simulink model "Requirement_table_and_model"  (R2022b)
settings: Solver=FixedStepAuto  StartTime=0.0  StopTime=10.0  FixedStep=1e-3  RelTol=1e-3  EnableMultiTasking=on
model workspace (MAT data in the model file):
  ATR_CMP_DETECT = canlib.Parameter
  ATR_CMP_DETECT.DataType = 'boolean'
  ATR_CMP_DETECT.Complexity = 'real'
  ATR_CMP_DETECT.Dimensions = [0 0]
  ATR_GND_CTRL = canlib.Parameter
  ATR_GND_CTRL.DataType = 'auto'
  ATR_GND_CTRL.Complexity = 'real'
  ATR_GND_CTRL.Dimensions = [0 0]
  ATR_PACE_CTRL = SimulinkDemos.Signal
  ATR_PACE_CTRL.DataType = 'auto'
  ATR_PACE_CTRL.Dimensions = -1
  ATR_PACE_CTRL.DimensionsMode = 'auto'
  ATR_PACE_CTRL.Complexity = 'auto'
  ATR_PACE_CTRL.SampleTime = -1
  ATR_PACE_CTRL.SamplingMode = 'auto'
  ATR_PULSE_WIDTH = SimulinkDemos.Signal
  ATR_PULSE_WIDTH.DataType = 'auto'
  ATR_PULSE_WIDTH.Dimensions = -1
  ATR_PULSE_WIDTH.DimensionsMode = 'auto'
  ATR_PULSE_WIDTH.Complexity = 'auto'
  ATR_PULSE_WIDTH.SampleTime = -1
  ATR_PULSE_WIDTH.SamplingMode = 'auto'
  ATR_REF = SimulinkDemos.Signal
  ATR_REF.DataType = 'auto'
  ATR_REF.Dimensions = -1
  ATR_REF.DimensionsMode = 'auto'
  ATR_REF.Complexity = 'auto'
  ATR_REF.SampleTime = -1
  ATR_REF.SamplingMode = 'auto'
  FRONTEND_CTRL = SimulinkDemos.Signal
  FRONTEND_CTRL.DataType = 'auto'
  FRONTEND_CTRL.Dimensions = -1
  FRONTEND_CTRL.DimensionsMode = 'auto'
  FRONTEND_CTRL.Complexity = 'auto'
  FRONTEND_CTRL.SampleTime = -1
  FRONTEND_CTRL.SamplingMode = 'auto'
  LRL = SimulinkDemos.Signal
  LRL.DataType = 'auto'
  LRL.Dimensions = -1
  LRL.DimensionsMode = 'auto'
  LRL.Complexity = 'auto'
  LRL.SampleTime = -1
  LRL.SamplingMode = 'auto'
  PACE_CHARGE_CTRL = SimulinkDemos.Signal
  PACE_CHARGE_CTRL.DataType = 'auto'
  PACE_CHARGE_CTRL.Dimensions = -1
  PACE_CHARGE_CTRL.DimensionsMode = 'auto'
  PACE_CHARGE_CTRL.Complexity = 'auto'
  PACE_CHARGE_CTRL.SampleTime = -1
  PACE_CHARGE_CTRL.SamplingMode = 'auto'
  PACE_GND_CTRL = SimulinkDemos.Signal
  PACE_GND_CTRL.DataType = 'auto'
  PACE_GND_CTRL.Dimensions = -1
  PACE_GND_CTRL.DimensionsMode = 'auto'
  PACE_GND_CTRL.Complexity = 'auto'
  PACE_GND_CTRL.SampleTime = -1
  PACE_GND_CTRL.SamplingMode = 'auto'
  VENT_CMP_DETECT = SimulinkDemos.Signal
  VENT_CMP_DETECT.DataType = 'auto'
  VENT_CMP_DETECT.Dimensions = -1
  VENT_CMP_DETECT.DimensionsMode = 'auto'
  VENT_CMP_DETECT.Complexity = 'auto'
  VENT_CMP_DETECT.SampleTime = -1
  VENT_CMP_DETECT.SamplingMode = 'auto'
  VENT_GND_CTRL = SimulinkDemos.Signal
  VENT_GND_CTRL.DataType = 'auto'
  VENT_GND_CTRL.Dimensions = -1
  VENT_GND_CTRL.DimensionsMode = 'auto'
  VENT_GND_CTRL.Complexity = 'auto'
  VENT_GND_CTRL.SampleTime = -1
  VENT_GND_CTRL.SamplingMode = 'auto'
  VENT_PACE_CTRL = SimulinkDemos.Signal
  VENT_PACE_CTRL.DataType = 'auto'
  VENT_PACE_CTRL.Dimensions = -1
  VENT_PACE_CTRL.DimensionsMode = 'auto'
  VENT_PACE_CTRL.Complexity = 'auto'
  VENT_PACE_CTRL.SampleTime = -1
  VENT_PACE_CTRL.SamplingMode = 'auto'
  VENT_PULSE_WIDTH = SimulinkDemos.Signal
  VENT_PULSE_WIDTH.DataType = 'auto'
  VENT_PULSE_WIDTH.Dimensions = -1
  VENT_PULSE_WIDTH.DimensionsMode = 'auto'
  VENT_PULSE_WIDTH.Complexity = 'auto'
  VENT_PULSE_WIDTH.SampleTime = -1
  VENT_PULSE_WIDTH.SamplingMode = 'auto'
  VENT_REF = SimulinkDemos.Signal
  VENT_REF.DataType = 'auto'
  VENT_REF.Dimensions = -1
  VENT_REF.DimensionsMode = 'auto'
  VENT_REF.Complexity = 'auto'
  VENT_REF.SampleTime = -1
  VENT_REF.SamplingMode = 'auto'
  Z_ATR_CTRL = SimulinkDemos.Signal
  Z_ATR_CTRL.DataType = 'auto'
  Z_ATR_CTRL.Dimensions = -1
  Z_ATR_CTRL.DimensionsMode = 'auto'
  Z_ATR_CTRL.Complexity = 'auto'
  Z_ATR_CTRL.SampleTime = -1
  Z_ATR_CTRL.SamplingMode = 'auto'
  Z_VENT_CTRL = SimulinkDemos.Signal
  Z_VENT_CTRL.DataType = 'auto'
  Z_VENT_CTRL.Dimensions = -1
  Z_VENT_CTRL.DimensionsMode = 'auto'
  Z_VENT_CTRL.Complexity = 'auto'
  Z_VENT_CTRL.SampleTime = -1
  Z_VENT_CTRL.SamplingMode = 'auto'
undefined symbols (not defined in the file): D0, D1, D10, D11, D12, D13, D2, D3, D4, D5, D6, D7, D8, D9, PTA0, PTA1, PTA2, PTB23, PTB9, PTC16, PTC17, PTC2, PTC3, PTC4, PTD0, PTD1, PTD2, PTD3
libraries: frdmk64flib x14
settings Model: ExtModeTrigDuration=5  Creator=clara  LastModifiedBy=dinghao
settings OptimizationCC: EnhancedBackFolding=on  PassReuseOutputArgsAs=Individual arguments  ZeroExternalMemoryAtStartup=off  ZeroInternalMemoryAtStartup=off  MaxStackSize=64  OptimizeBlockOrder=speed  DifferentSizesBufferReuse=on  OptimizationCustomize=off  EfficientTunableParamExpr=on
settings DebuggingCC: ParameterTunabilityLossMsg=error  SFUnusedDataAndEventsDiag=none
settings HardwareCC: ProdBitPerPointer=32  ProdBitPerSizeT=32  ProdBitPerPtrDiffT=32  ProdLargestAtomicInteger=Long  ProdLargestAtomicFloat=Double  ProdWordSize=32  ProdHWDeviceType=ARM Compatible->ARM Cortex
settings ModelReferenceCC: EnableRefExpFcnMdlSchedulingChecks=on
settings SFSimCC: MATLABDynamicMemAlloc=off
settings RTWCC: Description=Embedded Coder  SystemTargetFile=ert.tlc  HardwareBoard=NXP FRDM-K64F  TLCOptions="-aInlineSetEventsForThisBaseRateFcn=TLC_FALSE -aSuppressMultiTaskScheduler=TLC_FALSE  -aRateBasedStepFcn=0"  TemplateMakefile=ert_default_tmf  Toolchain=GNU Tools for ARM Embedded Processors
settings CodeAppCC: ForceParamTrailComments=on  IgnoreCustomStorageClasses=off  OperatorAnnotations=on  SimulinkDataObjDesc=on  SFDataObjDesc=on  InsertBlockDesc=on
settings ERTTargetCC: ExtModeTransport=4  ExtModeMexFile=sendToCommService

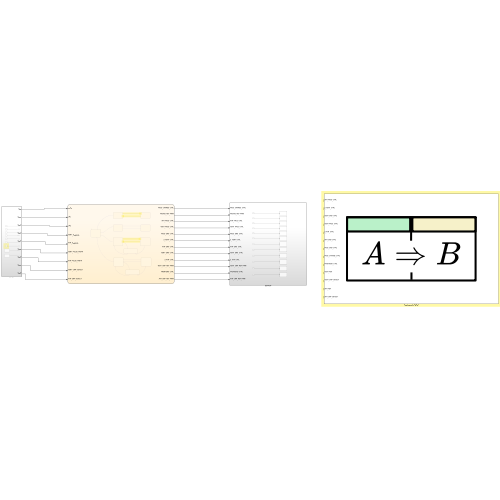
[thumbnail: Simulink's stored preview of the top-level diagram]
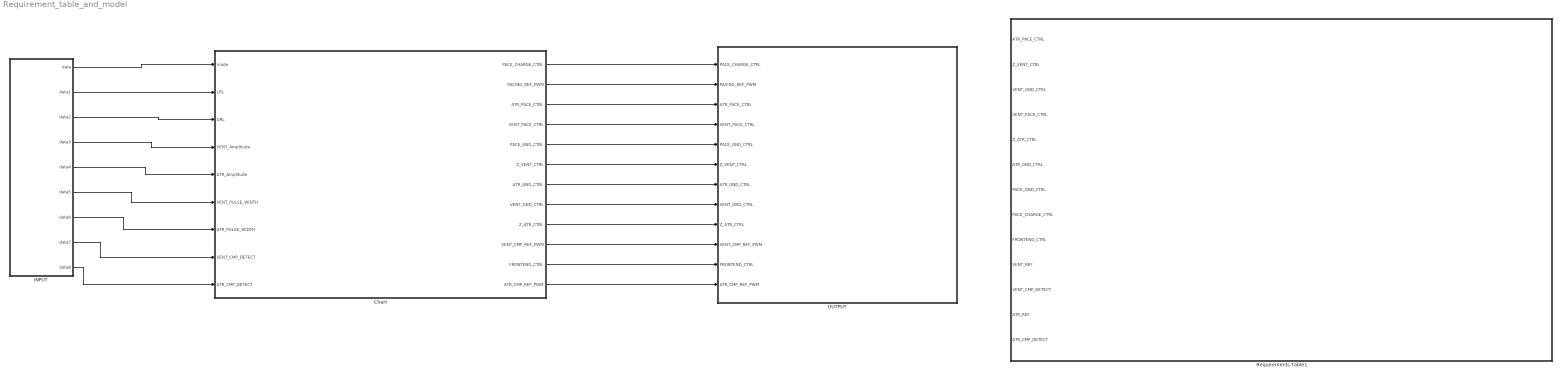
== system Requirement_table_and_model ==
  Chart : Stateflow chart  TreatAsAtomicUnit=on
      settings: PortSchema="{\"entries\":[{\"content\":{\"sides\":[{\"content\":{\"connectorIds\":[\"In9\",\"In1\",\"In6\",\"In2\",\"In3\",\"In4\",\"In5\",\"In7\",\"In8\"]},\"type\":\"ConnectorPlacement.EquallySpacedRectSide\",\"uuid\":\"411cfc43-89c3-4653-9fab-0da98be593d3\"},{\"content\":{\"connectorIds\":[\"Out1\",\"Out2\",\"Out3\",\"Out4\",\"Out5\",\"Out6\",\"Out7\",\"Out8\",\"Out9\",\"Out10\",\"Out11\",\"Out12\"],\"side\":\"RIGHT\"},\"type\":\"ConnectorPlacement.EquallySpacedRectSide\",\"uuid\":\"ad1683f7-26aa-4767-b656-f3b731cb8235\"},{\"content\":{\"connectorIds\":[],\"side\":\"TOP\"},\"type\":\"ConnectorPlacement.EquallySpacedRectSide\",\"uuid\":\"fbccba07-c1cc-4c9f-8e56-0bdfb6912bb8\"},{\"content\":{\"connectorIds\":[],\"side\":\"BOTTOM\"},\"type\":\"ConnectorPlacement.EquallySpacedRectSide\",\"uuid\":\"36d5a70a-9c4d-4c73-b058-58220445b1e8\"}]},\"type\":\"ConnectorPlacement.EquallySpacedConnector\",\"uuid\":\"0c618a7f-9484-4de3-a6ac-3c8308721375\"}],\"packageUris\":[\"http://schema.mathworks.com/mf0/Connector/R2020b\"],\"version\":\"1.0\"}"
  "INPUT " : Subsystem
  OUTPUT : Subsystem
  Requirements Table1 : Requirements Table  TreatAsAtomicUnit=on
  wires:
  Chart/7(ATR_GND_CTRL) -> OUTPUT/7(ATR_GND_CTRL)
  Chart/3(ATR_PACE_CTRL) -> OUTPUT/3(ATR_PACE_CTRL)
  Chart/6(Z_VENT_CTRL) -> OUTPUT/6(Z_VENT_CTRL)
  Chart/8(VENT_GND_CTRL) -> OUTPUT/8(VENT_GND_CTRL)
  Chart/5(PACE_GND_CTRL) -> OUTPUT/5(PACE_GND_CTRL)
  Chart/9(Z_ATR_CTRL) -> OUTPUT/9(Z_ATR_CTRL)
  Chart/2(PACING_REF_PWM) -> OUTPUT/2(PACING_REF_PWM)
  Chart/1(PACE_CHARGE_CTRL) -> OUTPUT/1(PACE_CHARGE_CTRL)
  Chart/4(VENT_PACE_CTRL) -> OUTPUT/4(VENT_PACE_CTRL)
  Chart/11(FRONTEND_CTRL) -> OUTPUT/11(FRONTEND_CTRL)
  Chart/10(VENT_CMP_REF_PWM) -> OUTPUT/10(VENT_CMP_REF_PWM)
  "INPUT "/1(data) -> Chart/9(mode)
  "INPUT "/3(data2) -> Chart/6(URL)
  "INPUT "/4(data3) -> Chart/2(VENT_Amplitude)
  "INPUT "/5(data4) -> Chart/3(ATR_Amplitude)
  "INPUT "/6(data5) -> Chart/4(VENT_PULSE_WIDTH)
  "INPUT "/8(data7) -> Chart/7(VENT_CMP_DETECT)
  Chart/12(ATR_CMP_REF_PWM) -> OUTPUT/12(ATR_CMP_REF_PWM)
  "INPUT "/7(data6) -> Chart/5(ATR_PULSE_WIDTH)
  "INPUT "/2(data1) -> Chart/1(LRL)
  "INPUT "/9(data8) -> Chart/8(ATR_CMP_DETECT)

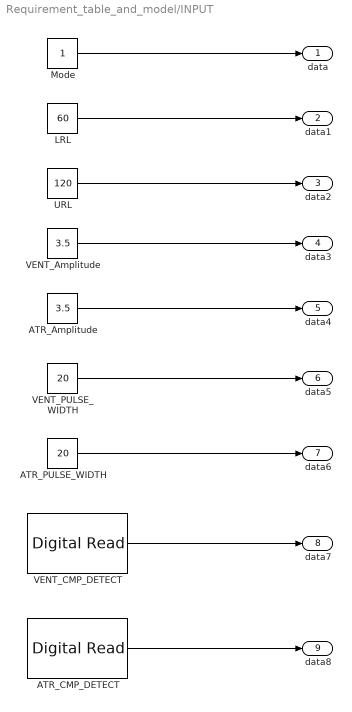
== system Requirement_table_and_model/INPUT  ==
  ATR_Amplitude : Constant  Value=3.5
  ATR_CMP_DETECT : frdmk64flib/Digital Read  Whichpin=PTC16 (D0)  SampleTime=-1
  ATR_PULSE_WIDTH : Constant  Value=20
  LRL : Constant  Value=60
  Mode : Constant
  URL : Constant  Value=120
  VENT_Amplitude : Constant  Value=3.5
  VENT_CMP_DETECT : frdmk64flib/Digital Read  Whichpin=PTC17 (D1)  SampleTime=-1
  VENT_PULSE_WIDTH : Constant  Value=20
  data : Outport
  data1 : Outport  Port=2
  data2 : Outport  Port=3
  data3 : Outport  Port=4
  data4 : Outport  Port=5
  data5 : Outport  Port=6
  data6 : Outport  Port=7
  data7 : Outport  Port=8
  data8 : Outport  Port=9
  wires:
  LRL/1 -> data1/1
  VENT_PULSE_WIDTH/1 -> data5/1
  VENT_Amplitude/1 -> data3/1
  URL/1 -> data2/1
  Mode/1 -> data/1
  ATR_Amplitude/1 -> data4/1
  ATR_PULSE_WIDTH/1 -> data6/1
  VENT_CMP_DETECT/1 -> data7/1
  ATR_CMP_DETECT/1 -> data8/1

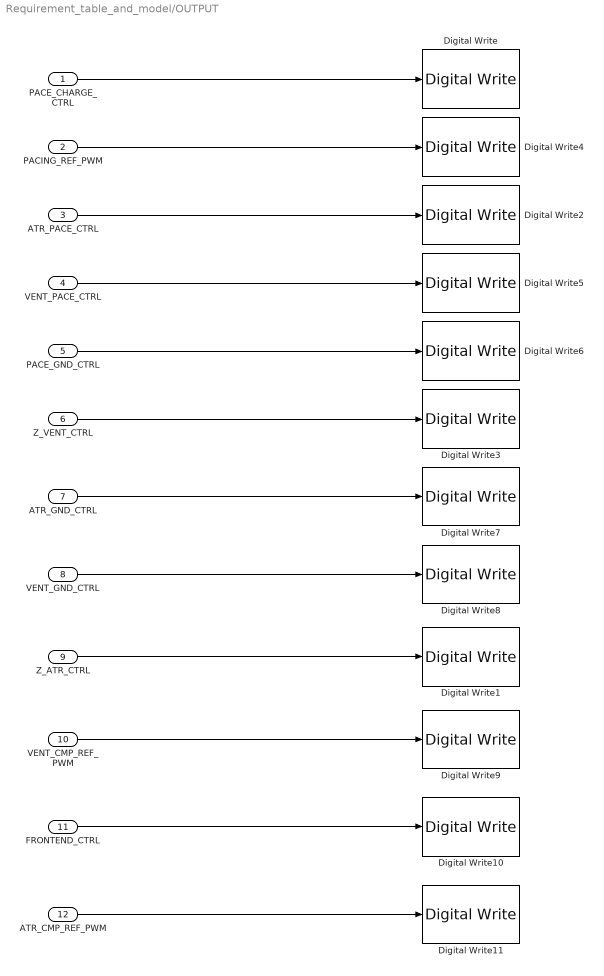
== system Requirement_table_and_model/OUTPUT ==
  PACE_CHARGE_CTRL : Inport
  PACING_REF_PWM : Inport  Port=2
  ATR_PACE_CTRL : Inport  Port=3
  VENT_PACE_CTRL : Inport  Port=4
  PACE_GND_CTRL : Inport  Port=5
  Z_VENT_CTRL : Inport  Port=6
  ATR_GND_CTRL : Inport  Port=7
  VENT_GND_CTRL : Inport  Port=8
  Z_ATR_CTRL : Inport  Port=9
  VENT_CMP_REF_PWM : Inport  Port=10
  FRONTEND_CTRL : Inport  Port=11
  ATR_CMP_REF_PWM : Inport  Port=12
  Digital Write : frdmk64flib/Digital Write  Whichpin=PTB9 (D2)
  Digital Write1 : frdmk64flib/Digital Write  Whichpin=PTB23 (D4)
  Digital Write10 : frdmk64flib/Digital Write  Whichpin=PTD1 (D13)
  Digital Write11 : frdmk64flib/Digital Write  Whichpin=PTC2 (D6)
  Digital Write2 : frdmk64flib/Digital Write  Whichpin=PTA0 (D8)
  Digital Write3 : frdmk64flib/Digital Write  Whichpin=PTC3 (D7)
  Digital Write4 : frdmk64flib/Digital Write  Whichpin=PTA2 (D5)
  Digital Write5 : frdmk64flib/Digital Write  Whichpin=PTC4 (D9)
  Digital Write6 : frdmk64flib/Digital Write  Whichpin=PTD0 (D10)
  Digital Write7 : frdmk64flib/Digital Write  Whichpin=PTD2 (D11)
  Digital Write8 : frdmk64flib/Digital Write  Whichpin=PTD3 (D12)
  Digital Write9 : frdmk64flib/Digital Write  Whichpin=PTA1 (D3)
  wires:
  PACE_CHARGE_CTRL/1 -> Digital Write/1
  PACING_REF_PWM/1 -> Digital Write4/1
  ATR_PACE_CTRL/1 -> Digital Write2/1
  VENT_PACE_CTRL/1 -> Digital Write5/1
  PACE_GND_CTRL/1 -> Digital Write6/1
  Z_VENT_CTRL/1 -> Digital Write3/1
  ATR_GND_CTRL/1 -> Digital Write7/1
  VENT_GND_CTRL/1 -> Digital Write8/1
  Z_ATR_CTRL/1 -> Digital Write1/1
  VENT_CMP_REF_PWM/1 -> Digital Write9/1
  FRONTEND_CTRL/1 -> Digital Write10/1
  ATR_CMP_REF_PWM/1 -> Digital Write11/1

== stateflow chart Requirement_table_and_model/Requirements Table1 ==
  (default) -> (junction 1073753366)
  (junction 1073753366) -> (junction 1073753367) : {
      | % SF_REQ_REV_07
      | }
  (junction 1073753367) -> (junction 1073753369) : {
      | % HEADER_ASSIGNMENTS
      |
      | }
  (junction 1073753369) -> (junction 1073753371) : {
      | % START_A_4
      | }
  (junction 1073753371) -> (junction 1073753373) : {
      | }
  (junction 1073753373) -> (junction 1073753375)
  (junction 1073753375) -> (junction 1073753377) : {
      | }
  (junction 1073753377) -> (junction 1073753379) : {
      | % END_A_4
      | }
  (junction 1073753379) -> (junction 1073753381) : {
      | % START_R_1
      | }
  (junction 1073753381) -> (junction 1073753383) : {
      | }
  (junction 1073753383) -> (junction 1073753385) : {
      |
      |
      |
      |
      |
      |
      |
      | }
  (junction 1073753385) -> (junction 1073753387) : {
      | }
  (junction 1073753387) -> (junction 1073753389) : {
      | % START_R_10
      | }
  (junction 1073753389) -> (junction 1073753391) : {
      | }
  (junction 1073753391) -> (junction 1073753393)
  (junction 1073753393) -> (junction 1073753395) [order 1] : [duration((prev(ATR_PACE_CTRL) == false) && (prev(PACE_CHARGE_CTRL) == true) && (prev(PACE_GND_CTRL) == true) && (prev(ATR_GND_CTRL) == true) && (prev(Z_ATR_CTRL) == false)) >= 60000/LRL-ATR_PULSE_WIDTH]
  (junction 1073753393) -> (junction 1073753401) [order 2]
  (junction 1073753395) -> (junction 1073753397) : {
      | ATR_PACE_CTRL == true
      | PACE_CHARGE_CTRL == false
      | PACE_GND_CTRL == true
      | ATR_GND_CTRL == false
      | Z_ATR_CTRL == false
      |
      |
      | }
  (junction 1073753397) -> (junction 1073753399) : {
      | }
  (junction 1073753399) -> (junction 1073753401)
  (junction 1073753401) -> (junction 1073753403)
  (junction 1073753403) -> (junction 1073753405) : {
      | % END_R_10
      | }
  (junction 1073753405) -> (junction 1073753407) : {
      | % START_R_13
      | }
  (junction 1073753407) -> (junction 1073753409) : {
      | }
  (junction 1073753409) -> (junction 1073753411)
  (junction 1073753411) -> (junction 1073753413) [order 1] : [duration((prev(ATR_PACE_CTRL) == true) && (prev(PACE_CHARGE_CTRL)== false) && (prev(PACE_GND_CTRL) == true) && (prev(ATR_GND_CTRL) == false) && (prev(Z_ATR_CTRL) == false)) >= ATR_PULSE_WIDTH]
  (junction 1073753411) -> (junction 1073753419) [order 2]
  (junction 1073753413) -> (junction 1073753415) : {
      | ATR_PACE_CTRL == false
      | PACE_CHARGE_CTRL == true
      | PACE_GND_CTRL == true
      | ATR_GND_CTRL == true
      | Z_ATR_CTRL == false
      |
      |
      | }
  (junction 1073753415) -> (junction 1073753417) : {
      | }
  (junction 1073753417) -> (junction 1073753419)
  (junction 1073753419) -> (junction 1073753421)
  (junction 1073753421) -> (junction 1073753423) : {
      | % END_R_13
      | }
  (junction 1073753423) -> (junction 1073753425) : {
      | % END_R_1
      | }
  (junction 1073753425) -> (junction 1073753427) : {
      | % START_R_16
      | }
  (junction 1073753427) -> (junction 1073753429) : {
      | }
  (junction 1073753429) -> (junction 1073753431) : {
      |
      |
      |
      |
      |
      |
      |
      | }
  (junction 1073753431) -> (junction 1073753433) : {
      | }
  (junction 1073753433) -> (junction 1073753435) : {
      | % START_R_19
      | }
  (junction 1073753435) -> (junction 1073753437) : {
      | }
  (junction 1073753437) -> (junction 1073753439)
  (junction 1073753439) -> (junction 1073753441) [order 1] : [duration((prev(VENT_PACE_CTRL) == false) && (prev(PACE_CHARGE_CTRL) == true) && (prev(VENT_GND_CTRL) == true) && (prev(PACE_GND_CTRL) == true) && (prev(Z_VENT_CTRL) == false)) >= 60000/LRL-VENT_PULSE_WIDTH]
  (junction 1073753439) -> (junction 1073753447) [order 2]
  (junction 1073753441) -> (junction 1073753443) : {
      | VENT_PACE_CTRL == true
      | PACE_CHARGE_CTRL == false
      | VENT_GND_CTRL == false
      | PACE_GND_CTRL == true
      | Z_VENT_CTRL == false
      |
      |
      | }
  (junction 1073753443) -> (junction 1073753445) : {
      | }
  (junction 1073753445) -> (junction 1073753447)
  (junction 1073753447) -> (junction 1073753449)
  (junction 1073753449) -> (junction 1073753451) : {
      | % END_R_19
      | }
  (junction 1073753451) -> (junction 1073753453) : {
      | % START_R_22
      | }
  (junction 1073753453) -> (junction 1073753455) : {
      | }
  (junction 1073753455) -> (junction 1073753457)
  (junction 1073753457) -> (junction 1073753459) [order 1] : [duration((prev(VENT_PACE_CTRL) == true) && (prev(PACE_CHARGE_CTRL) == false) && (prev(VENT_GND_CTRL) == false) && (prev(PACE_GND_CTRL) == true) && (prev(Z_VENT_CTRL) == false)) >= VENT_PULSE_WIDTH]
  (junction 1073753457) -> (junction 1073753465) [order 2]
  (junction 1073753459) -> (junction 1073753461) : {
      | VENT_PACE_CTRL == false
      | PACE_CHARGE_CTRL == true
      | VENT_GND_CTRL == true
      | PACE_GND_CTRL == true
      | Z_VENT_CTRL == false
      |
      |
      | }
  (junction 1073753461) -> (junction 1073753463) : {
      | }
  (junction 1073753463) -> (junction 1073753465)
  (junction 1073753465) -> (junction 1073753467)
  (junction 1073753467) -> (junction 1073753469) : {
      | % END_R_22
      | }
  (junction 1073753469) -> (junction 1073753471) : {
      | % END_R_16
      | }
  (junction 1073753471) -> (junction 1073753473) : {
      | % START_R_25
      | }
  (junction 1073753473) -> (junction 1073753475) : {
      | }
  (junction 1073753475) -> (junction 1073753477) : {
      |
      |
      |
      |
      |
      |
      |
      | }
  (junction 1073753477) -> (junction 1073753479) : {
      | }
  (junction 1073753479) -> (junction 1073753481) : {
      | % START_R_28
      | }
  (junction 1073753481) -> (junction 1073753483) : {
      | }
  (junction 1073753483) -> (junction 1073753485)
  (junction 1073753485) -> (junction 1073753487) [order 1] : [(prev(FRONTEND_CTRL) == true ) && (prev(VENT_PACE_CTRL) == false) && (prev(PACE_CHARGE_CTRL) == true) && (prev(PACE_GND_CTRL) == true) && (prev(VENT_GND_CTRL) == true) && (prev(Z_VENT_CTRL) == false)]
  (junction 1073753485) -> (junction 1073753529) [order 2]
  (junction 1073753487) -> (junction 1073753489) : {
      |
      |
      |
      |
      |
      |
      |
      | }
  (junction 1073753489) -> (junction 1073753491) : {
      | }
  (junction 1073753491) -> (junction 1073753493) : {
      | % START_R_49
      | }
  (junction 1073753493) -> (junction 1073753495) : {
      | }
  (junction 1073753495) -> (junction 1073753497)
  (junction 1073753497) -> (junction 1073753499) [order 1] : [(prev(VENT_CMP_DETECT) == true)]
  (junction 1073753497) -> (junction 1073753505) [order 2]
  (junction 1073753499) -> (junction 1073753501) : {
      | (FRONTEND_CTRL) == false
      | (VENT_PACE_CTRL) == false
      | (PACE_CHARGE_CTRL) == true
      | (PACE_GND_CTRL) == true
      | (VENT_GND_CTRL) == true
      | (Z_VENT_CTRL) == false
      |
      | }
  (junction 1073753501) -> (junction 1073753503) : {
      | }
  (junction 1073753503) -> (junction 1073753505)
  (junction 1073753505) -> (junction 1073753507)
  (junction 1073753507) -> (junction 1073753509) : {
      | % END_R_49
      | }
  (junction 1073753509) -> (junction 1073753511) : {
      | % START_R_52
      | }
  (junction 1073753511) -> (junction 1073753513) : {
      | }
  (junction 1073753513) -> (junction 1073753515)
  (junction 1073753515) -> (junction 1073753517) [order 1] : [duration((prev(VENT_CMP_DETECT) == false)) >= 60000/LRL-VENT_PULSE_WIDTH]
  (junction 1073753515) -> (junction 1073753523) [order 2]
  (junction 1073753517) -> (junction 1073753519) : {
      | (FRONTEND_CTRL) == true
      | (VENT_PACE_CTRL) == true
      | (PACE_CHARGE_CTRL) == false
      | (PACE_GND_CTRL) == true
      | (VENT_GND_CTRL) == false
      | (Z_VENT_CTRL) == false
      |
      | }
  (junction 1073753519) -> (junction 1073753521) : {
      | }
  (junction 1073753521) -> (junction 1073753523)
  (junction 1073753523) -> (junction 1073753525)
  (junction 1073753525) -> (junction 1073753527) : {
      | % END_R_52
      | }
  (junction 1073753527) -> (junction 1073753529)
  (junction 1073753529) -> (junction 1073753531)
  (junction 1073753531) -> (junction 1073753533) : {
      | % END_R_28
      | }
  (junction 1073753533) -> (junction 1073753535) : {
      | % START_R_31
      | }
  (junction 1073753535) -> (junction 1073753537) : {
      | }
  (junction 1073753537) -> (junction 1073753539)
  (junction 1073753539) -> (junction 1073753541) [order 1] : [duration((prev(FRONTEND_CTRL) == true ) && (prev(VENT_PACE_CTRL) == true) && (prev(PACE_CHARGE_CTRL) == false) && (prev(PACE_GND_CTRL) == true) && (prev(VENT_GND_CTRL) == false) && (prev(Z_VENT_CTRL) == false)) >= VENT_PULSE_WIDTH]
  (junction 1073753539) -> (junction 1073753583) [order 2]
  (junction 1073753541) -> (junction 1073753543) : {
      |
      |
      |
      |
      |
      |
      |
      | }
  (junction 1073753543) -> (junction 1073753545) : {
      | }
  (junction 1073753545) -> (junction 1073753547) : {
      | % START_R_55
      | }
  (junction 1073753547) -> (junction 1073753549) : {
      | }
  (junction 1073753549) -> (junction 1073753551)
  (junction 1073753551) -> (junction 1073753553) [order 1] : [(prev(VENT_CMP_DETECT) == true)]
  (junction 1073753551) -> (junction 1073753559) [order 2]
  (junction 1073753553) -> (junction 1073753555) : {
      | (FRONTEND_CTRL) == false
      | (VENT_PACE_CTRL) == false
      | (PACE_CHARGE_CTRL) == true
      | (PACE_GND_CTRL) == true
      | (VENT_GND_CTRL) == true
      | (Z_VENT_CTRL) == false
      |
      | }
  (junction 1073753555) -> (junction 1073753557) : {
      | }
  (junction 1073753557) -> (junction 1073753559)
  (junction 1073753559) -> (junction 1073753561)
  (junction 1073753561) -> (junction 1073753563) : {
      | % END_R_55
      | }
  (junction 1073753563) -> (junction 1073753565) : {
      | % START_R_58
      | }
  (junction 1073753565) -> (junction 1073753567) : {
      | }
  (junction 1073753567) -> (junction 1073753569)
  (junction 1073753569) -> (junction 1073753571) [order 1] : [(prev(VENT_CMP_DETECT) == false)]
  (junction 1073753569) -> (junction 1073753577) [order 2]
  (junction 1073753571) -> (junction 1073753573) : {
      | (FRONTEND_CTRL) == true
      | (VENT_PACE_CTRL) == false
      | (PACE_CHARGE_CTRL) == true
      | (PACE_GND_CTRL) == true
      | (VENT_GND_CTRL) == true
      | (Z_VENT_CTRL) == false
      |
      | }
  (junction 1073753573) -> (junction 1073753575) : {
      | }
  (junction 1073753575) -> (junction 1073753577)
  (junction 1073753577) -> (junction 1073753579)
  (junction 1073753579) -> (junction 1073753581) : {
      | % END_R_58
      | }
  (junction 1073753581) -> (junction 1073753583)
  (junction 1073753583) -> (junction 1073753585)
  (junction 1073753585) -> (junction 1073753587) : {
      | % END_R_31
      | }
  (junction 1073753587) -> (junction 1073753589) : {
      | % START_R_34
      | }
  (junction 1073753589) -> (junction 1073753591) : {
      | }
  (junction 1073753591) -> (junction 1073753593)
  (junction 1073753593) -> (junction 1073753595) [order 1] : [(prev(FRONTEND_CTRL) == false) && (prev(VENT_PACE_CTRL) == false) && (prev(PACE_CHARGE_CTRL) == true) && (prev(PACE_GND_CTRL) == true) && (prev(VENT_GND_CTRL) == true) && (prev(Z_VENT_CTRL) == false)]
  (junction 1073753593) -> (junction 1073753601) [order 2]
  (junction 1073753595) -> (junction 1073753597) : {
      | (FRONTEND_CTRL) == true
      | (VENT_PACE_CTRL) == false
      | (PACE_CHARGE_CTRL) == true
      | (PACE_GND_CTRL) == true
      | (VENT_GND_CTRL) == true
      | (Z_VENT_CTRL) == false
      |
      | }
  (junction 1073753597) -> (junction 1073753599) : {
      | }
  (junction 1073753599) -> (junction 1073753601)
  (junction 1073753601) -> (junction 1073753603)
  (junction 1073753603) -> (junction 1073753605) : {
      | % END_R_34
      | }
  (junction 1073753605) -> (junction 1073753607) : {
      | % END_R_25
      | }
  (junction 1073753607) -> (junction 1073753609) : {
      | % START_R_37
      | }
  (junction 1073753609) -> (junction 1073753611) : {
      | }
  (junction 1073753611) -> (junction 1073753613) : {
      |
      |
      |
      |
      |
      |
      |
      | }
  (junction 1073753613) -> (junction 1073753615) : {
      | }
  (junction 1073753615) -> (junction 1073753617) : {
      | % START_R_40
      | }
  (junction 1073753617) -> (junction 1073753619) : {
      | }
  (junction 1073753619) -> (junction 1073753621)
  (junction 1073753621) -> (junction 1073753623) [order 1] : [(prev(FRONTEND_CTRL) == true ) && (prev(ATR_PACE_CTRL) == false) && (prev(PACE_CHARGE_CTRL) == true) && (prev(PACE_GND_CTRL) == true) && (prev(ATR_GND_CTRL) == true) && (prev(Z_ATR_CTRL) == false)]
  (junction 1073753621) -> (junction 1073753665) [order 2]
  (junction 1073753623) -> (junction 1073753625) : {
      |
      |
      |
      |
      |
      |
      |
      | }
  (junction 1073753625) -> (junction 1073753627) : {
      | }
  (junction 1073753627) -> (junction 1073753629) : {
      | % START_R_61
      | }
  (junction 1073753629) -> (junction 1073753631) : {
      | }
  (junction 1073753631) -> (junction 1073753633)
  (junction 1073753633) -> (junction 1073753635) [order 1] : [(prev(ATR_CMP_DETECT) == true)]
  (junction 1073753633) -> (junction 1073753641) [order 2]
  (junction 1073753635) -> (junction 1073753637) : {
      | (FRONTEND_CTRL) == false
      | (ATR_PACE_CTRL) == false
      | (PACE_CHARGE_CTRL) == true
      | (PACE_GND_CTRL) == true
      | (ATR_GND_CTRL) == true
      | (Z_ATR_CTRL) == false
      |
      | }
  (junction 1073753637) -> (junction 1073753639) : {
      | }
  (junction 1073753639) -> (junction 1073753641)
  (junction 1073753641) -> (junction 1073753643)
  (junction 1073753643) -> (junction 1073753645) : {
      | % END_R_61
      | }
  (junction 1073753645) -> (junction 1073753647) : {
      | % START_R_64
      | }
  (junction 1073753647) -> (junction 1073753649) : {
      | }
  (junction 1073753649) -> (junction 1073753651)
  (junction 1073753651) -> (junction 1073753653) [order 1] : [duration((prev(ATR_CMP_DETECT) == false)) >= 60000/LRL-ATR_PULSE_WIDTH]
  (junction 1073753651) -> (junction 1073753659) [order 2]
  (junction 1073753653) -> (junction 1073753655) : {
      | (FRONTEND_CTRL) == true
      | (ATR_PACE_CTRL) == true
      | (PACE_CHARGE_CTRL) == false
      | (PACE_GND_CTRL) == true
      | (ATR_GND_CTRL) == false
      | (Z_ATR_CTRL) == false
      |
      | }
  (junction 1073753655) -> (junction 1073753657) : {
      | }
  (junction 1073753657) -> (junction 1073753659)
  (junction 1073753659) -> (junction 1073753661)
  (junction 1073753661) -> (junction 1073753663) : {
      | % END_R_64
      | }
  (junction 1073753663) -> (junction 1073753665)
  (junction 1073753665) -> (junction 1073753667)
  (junction 1073753667) -> (junction 1073753669) : {
      | % END_R_40
      | }
  (junction 1073753669) -> (junction 1073753671) : {
      | % START_R_43
      | }
  (junction 1073753671) -> (junction 1073753673) : {
      | }
  (junction 1073753673) -> (junction 1073753675)
  (junction 1073753675) -> (junction 1073753677) [order 1] : [duration((prev(FRONTEND_CTRL) == true ) && (prev(ATR_PACE_CTRL) == true) && (prev(PACE_CHARGE_CTRL) == false) && (prev(PACE_GND_CTRL) == true) && (prev(ATR_GND_CTRL) == false) && (prev(Z_ATR_CTRL) == false)) >= ATR_PULSE_WIDTH]
  (junction 1073753675) -> (junction 1073753719) [order 2]
  (junction 1073753677) -> (junction 1073753679) : {
      |
      |
      |
      |
      |
      |
      |
      | }
  (junction 1073753679) -> (junction 1073753681) : {
      | }
  (junction 1073753681) -> (junction 1073753683) : {
      | % START_R_67
      | }
  (junction 1073753683) -> (junction 1073753685) : {
      | }
  (junction 1073753685) -> (junction 1073753687)
  (junction 1073753687) -> (junction 1073753689) [order 1] : [(prev(VENT_CMP_DETECT) == true)]
  (junction 1073753687) -> (junction 1073753695) [order 2]
  (junction 1073753689) -> (junction 1073753691) : {
      | (FRONTEND_CTRL) == false
      | (ATR_PACE_CTRL) == false
      | (PACE_CHARGE_CTRL) == true
      | (PACE_GND_CTRL) == true
      | (ATR_GND_CTRL) == true
      | (Z_ATR_CTRL) == false
      |
      | }
  (junction 1073753691) -> (junction 1073753693) : {
      | }
  (junction 1073753693) -> (junction 1073753695)
  (junction 1073753695) -> (junction 1073753697)
  (junction 1073753697) -> (junction 1073753699) : {
      | % END_R_67
      | }
  (junction 1073753699) -> (junction 1073753701) : {
      | % START_R_70
      | }
  (junction 1073753701) -> (junction 1073753703) : {
      | }
  (junction 1073753703) -> (junction 1073753705)
  (junction 1073753705) -> (junction 1073753707) [order 1] : [(prev(VENT_CMP_DETECT) == false)]
  (junction 1073753705) -> (junction 1073753713) [order 2]
  (junction 1073753707) -> (junction 1073753709) : {
      | (FRONTEND_CTRL) == true
      | (ATR_PACE_CTRL) == false
      | (PACE_CHARGE_CTRL) == true
      | (PACE_GND_CTRL) == true
      | (ATR_GND_CTRL) == true
      | (Z_ATR_CTRL) == false
      |
      | }
  (junction 1073753709) -> (junction 1073753711) : {
      | }
  (junction 1073753711) -> (junction 1073753713)
  (junction 1073753713) -> (junction 1073753715)
  (junction 1073753715) -> (junction 1073753717) : {
      | % END_R_70
      | }
  (junction 1073753717) -> (junction 1073753719)
  (junction 1073753719) -> (junction 1073753721)
  (junction 1073753721) -> (junction 1073753723) : {
      | % END_R_43
      | }
  (junction 1073753723) -> (junction 1073753725) : {
      | % START_R_46
      | }
  (junction 1073753725) -> (junction 1073753727) : {
      | }
  (junction 1073753727) -> (junction 1073753729)
  (junction 1073753729) -> (junction 1073753731) [order 1] : [(prev(FRONTEND_CTRL) == false) && (prev(ATR_PACE_CTRL) == false) && (prev(PACE_CHARGE_CTRL) == true) && (prev(PACE_GND_CTRL) == true) && (prev(ATR_GND_CTRL) == true) && (prev(Z_ATR_CTRL) == false)]
  (junction 1073753729) -> (junction 1073753737) [order 2]
  (junction 1073753731) -> (junction 1073753733) : {
      | (FRONTEND_CTRL) == true
      | (ATR_PACE_CTRL) == false
      | (PACE_CHARGE_CTRL) == true
      | (PACE_GND_CTRL) == true
      | (ATR_GND_CTRL) == true
      | (Z_ATR_CTRL) == false
      |
      | }
  (junction 1073753733) -> (junction 1073753735) : {
      | }
  (junction 1073753735) -> (junction 1073753737)
  (junction 1073753737) -> (junction 1073753739)
  (junction 1073753739) -> (junction 1073753741) : {
      | % END_R_46
      | }
  (junction 1073753741) -> (junction 1073753743) : {
      | % END_R_37
      | }
  data: ATR_PACE_CTRL input boolean; Z_VENT_CTRL input boolean; VENT_GND_CTRL input boolean; VENT_PACE_CTRL input boolean; Z_ATR_CTRL input boolean; ATR_GND_CTRL input boolean; PACE_GND_CTRL input boolean; PACE_CHARGE_CTRL input boolean; FRONTEND_CTRL input boolean; VENT_REF input int8; VENT_CMP_DETECT input boolean; ATR_REF input int8; LRL constant int8; VENT_PULSE_WIDTH constant int8; ATR_PULSE_WIDTH constant int8; ATR_CMP_DETECT input boolean

== stateflow chart Requirement_table_and_model/Chart ==
  state AOO
    entry:
    % charge condition for C22
    ATR_PACE_CTRL = false;
    VENT_PACE_CTRL = false;
    PACE_CHARGE_CTRL = true;
    % discharge condition for C21;
    VENT_GND_CTRL = false;
    PACE_GND_CTRL = true;
    ATR_GND_CTRL = true;
    Z_ATR_CTRL = false;
    Z_VENT_CTRL = false;
    %
    PACING_REF_PWM = 20*ATR_Amplitude;
  state Pacing_AOO
    entry:
    PACE_CHARGE_CTRL = false;
    PACE_GND_CTRL = true;
    ATR_PACE_CTRL = true;
    ATR_GND_CTRL = false;
    Z_ATR_CTRL = false;
    Z_VENT_CTRL = false;
    VENT_GND_CTRL = false;
    VENT_PACE_CTRL = false;
    %
  state VOO
    entry:
    % charge condition for C22
    ATR_PACE_CTRL = false;
    VENT_PACE_CTRL = false;
    PACE_CHARGE_CTRL = true;
    % discharge condition for C21;
    VENT_GND_CTRL = true;
    PACE_GND_CTRL = true;
    ATR_GND_CTRL = false;
    Z_ATR_CTRL = false;
    Z_VENT_CTRL = false;
    %
    PACING_REF_PWM = 20*VENT_Amplitude;
  state Pacing_VOO
    entry:
    PACE_CHARGE_CTRL = false;
    PACE_GND_CTRL = true;
    ATR_PACE_CTRL = false;
    ATR_GND_CTRL = false;
    Z_ATR_CTRL = false;
    Z_VENT_CTRL = false;
    VENT_GND_CTRL = false;
    VENT_PACE_CTRL = true;
    %
  state MAIN
    entry:
    VENT_GND_CTRL=false;
    Z_ATR_CTRL = false;
    Z_VENT_CTRL = false;
    FRONTEND_CTRL=false;
    PACE_CHARGE_CTRL = false;
    VENT_PACE_CTRL = false;
    ATR_PACE_CTRL = false;
    PACE_GND_CTRL=false;
    ATR_GND_CTRL=false;
  state AAI
    entry:
    % begin sensing
    FRONTEND_CTRL = true;
    % charge condition for C22
    ATR_PACE_CTRL = false;
    VENT_PACE_CTRL = false;
    PACE_CHARGE_CTRL = true;
    % discharge condition for C21;
    ATR_GND_CTRL = true;
    PACE_GND_CTRL = true;
    VENT_GND_CTRL = false;
    Z_ATR_CTRL = false;
    Z_VENT_CTRL = false;
    %
    PACING_REF_PWM = 20*ATR_Amplitude;
    ATR_CMP_REF_PWM = 20*ATR_Amplitude;
  state Pacing_VVI1
    entry:
    PACE_CHARGE_CTRL = false;
    PACE_GND_CTRL = true;
    ATR_PACE_CTRL = true;
    ATR_GND_CTRL = false;
    Z_ATR_CTRL = false;
    Z_VENT_CTRL = false;
    VENT_GND_CTRL = false;
    VENT_PACE_CTRL = false;
    %
    PACING_REF_PWM = 20*ATR_Amplitude;
  state AAI_REFRACTORY
    entry:
    FRONTEND_CTRL = false;
    ATR_PACE_CTRL = false;
    VENT_PACE_CTRL = false;
    ATR_GND_CTRL = true;
    PACING_REF_PWM = 20*ATR_Amplitude;
    PACE_CHARGE_CTRL = false;
    PACE_GND_CTRL = true;
  state VVI
    entry:
    % begin sensing
    FRONTEND_CTRL = true;
    % charge condition for C22
    ATR_PACE_CTRL = false;
    VENT_PACE_CTRL = false;
    PACE_CHARGE_CTRL = true;
    % discharge condition for C21;
    VENT_GND_CTRL = true;
    PACE_GND_CTRL = true;
    ATR_GND_CTRL = false;
    Z_ATR_CTRL = false;
    Z_VENT_CTRL = false;
    %
    PACING_REF_PWM = 20*VENT_Amplitude;
    VENT_CMP_REF_PWM = 20*VENT_Amplitude;
  state Pacing_VVI
    entry:
    PACE_CHARGE_CTRL = false;
    PACE_GND_CTRL = true;
    ATR_PACE_CTRL = false;
    ATR_GND_CTRL = false;
    Z_ATR_CTRL = false;
    Z_VENT_CTRL = false;
    VENT_GND_CTRL = false;
    VENT_PACE_CTRL = true;
    %
    PACING_REF_PWM = 20*VENT_Amplitude;
  state VVI_REFRACTORY
    entry:
    FRONTEND_CTRL = false;
    ATR_PACE_CTRL = false;
    VENT_GND_CTRL = true;
    PACING_REF_PWM = 20*VENT_Amplitude;
    PACE_CHARGE_CTRL = false;
    PACE_GND_CTRL = true;
  AOO -> Pacing_AOO : [after(60000/LRL - ATR_PULSE_WIDTH,msec)]
  MAIN -> AOO [order 4] : [mode == 1]
  Pacing_AOO -> AOO : [after(ATR_PULSE_WIDTH,msec)]
  VOO -> Pacing_VOO : [after(60000/LRL - VENT_PULSE_WIDTH,msec)]
  MAIN -> VOO [order 1] : [mode == 2]
  (default) -> MAIN
  Pacing_VOO -> VOO : [after(VENT_PULSE_WIDTH,msec)]
  MAIN -> AAI [order 3] : [mode == 3]
  MAIN -> VVI [order 2] : [mode == 4]
  AAI -> Pacing_VVI1 [order 1] : [(ATR_CMP_DETECT==false) &&after(60000/LRL - ATR_PULSE_WIDTH,msec)]
  Pacing_VVI1 -> AAI [order 1] : [after(ATR_PULSE_WIDTH,msec)]
  AAI -> AAI_REFRACTORY [order 2] : [ATR_CMP_DETECT == true]
  AAI_REFRACTORY -> AAI
  Pacing_VVI1 -> AAI_REFRACTORY [order 2] : [ATR_CMP_DETECT == true]
  VVI -> Pacing_VVI [order 1] : [(VENT_CMP_DETECT==false) &&after(60000/LRL - VENT_PULSE_WIDTH,msec)]
  Pacing_VVI -> VVI [order 1] : [after(VENT_PULSE_WIDTH,msec)]
  VVI -> VVI_REFRACTORY [order 2] : [VENT_CMP_DETECT == true]
  VVI_REFRACTORY -> VVI
  Pacing_VVI -> VVI_REFRACTORY [order 2] : [VENT_CMP_DETECT == true]
  data: LRL input; VENT_Amplitude input; ATR_Amplitude input; VENT_PULSE_WIDTH input; ATR_PULSE_WIDTH input; URL input; VENT_CMP_DETECT input; ATR_CMP_DETECT input; PACE_CHARGE_CTRL output; PACING_REF_PWM output; ATR_PACE_CTRL output; VENT_PACE_CTRL output; PACE_GND_CTRL output; Z_VENT_CTRL output; ATR_GND_CTRL output; VENT_GND_CTRL output; Z_ATR_CTRL output; VENT_CMP_REF_PWM output; FRONTEND_CTRL output; mode input; ATR_CMP_REF_PWM output
